simulink model "scheme_w_Adaptive"  (R2025a)
settings: Solver=ode4  StartTime=0.0  StopTime=36  FixedStep=0.001  RelTol=1e-3
values from neighbouring files (symbols this model uses):
  x0 = zeros(14, 1)    [Planning_Sim.m]
undefined symbols (not defined in the file or in its folder): alpha, Am_x, Am_y, Am_z, B_pitch, B_roll, B_spin, beta, Bm_x, Bm_y, Bm_z, Cm_x, Cm_y, Dm_x, Dm_y, gamma, p, Px, Py, Pz
settings Model: Creator=chiar_zjcy1by  LastModifiedBy=chiar_zjcy1by
settings SolverCC: ZeroCrossAlgorithm=Adaptive
settings DebuggingCC: IgnoredZcDiagnostic=none

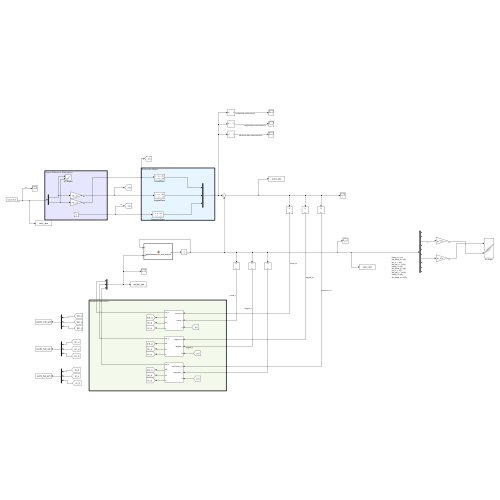
[thumbnail: Simulink's stored preview of the top-level diagram]
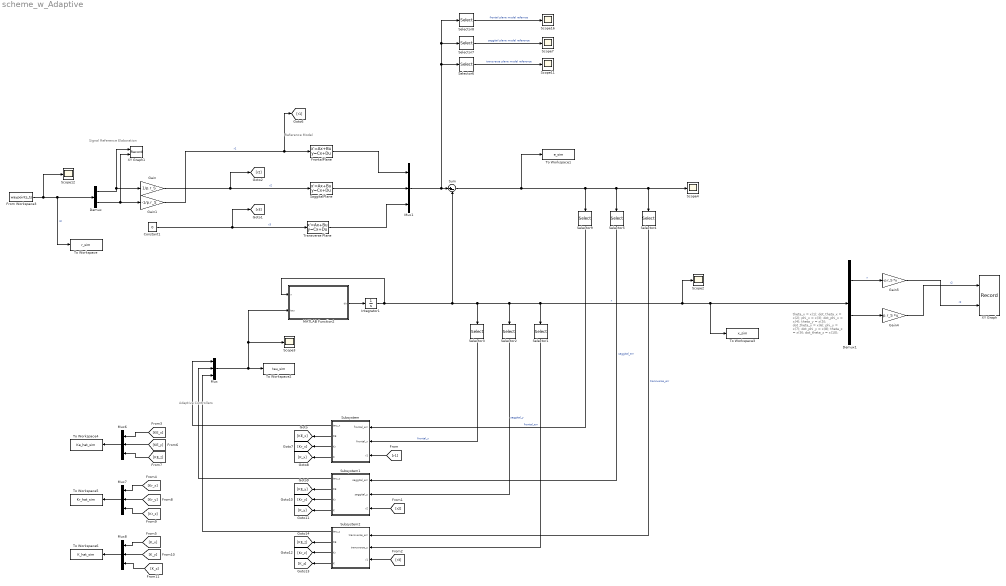
== system scheme_w_Adaptive ==
  note: Signal Reference Elaboration
  note: Reference Model
  note: Adaptive Controllers
  note: theta_x = x(1);
      | dot_theta_x = x(2);
      | phi_x = x(3);
      | dot_phi_x = x(4);
      | theta_y = x(5);
      | dot_theta_y = x(6);
      | phi_y = x(7);
      | dot_phi_y = x(8);
      | theta_z = x(9);
      | dot_theta_z = x(10);
  Constant1 : Constant  Value=0
  Demux : Demux  Outputs=2
  Demux1 : Demux  Outputs=10
  From Workspace3 : FromWorkspace  VariableName=waypoints_ts  SampleTime=0.01  OutputAfterFinalValue=Holding final value
  FrontalPlane : StateSpace  A=Am_x  B=Bm_x  C=Cm_x  D=Dm_x  InitialCondition=x0(1:4)
  Gain : Gain  Gain=1/p.r_S
  Gain1 : Gain  Gain=-1/p.r_S
  Gain4 : Gain  Gain=p.r_S  Multiplication=Matrix(K*u)
  Gain5 : Gain  Gain=-p.r_S  Multiplication=Matrix(K*u)
  Integrator1 : Integrator  InitialCondition=x0
  MATLAB Function2 : MATLAB Function  TreatAsAtomicUnit=on
  Mux{,1,6..8} (5 alike) : Mux  Inputs=3
  SaggitalPlane : StateSpace  A=Am_y  B=Bm_y  C=Cm_y  D=Dm_y  InitialCondition=x0(5:8)
  Scope{2..4,7,11..12,16} (7 alike) : Scope
      Scope11 settings: ActiveDisplayYMinimum=-1  ActiveDisplayYMaximum=1  DataLoggingVariableName=ScopeData19
      Scope12 settings: ActiveDisplayYMinimum=-0.55116650388768529  ActiveDisplayYMaximum=4.9604985349891688  DataLoggingVariableName=ScopeData20  DataLoggingSaveFormat=Array
      Scope16 settings: ActiveDisplayYMinimum=-1.561360729010373  ActiveDisplayYMaximum=5.3735398831765027  DataLoggingVariableName=ScopeData25
      Scope2 settings: ActiveDisplayYMinimum=-2.4855756069167088  ActiveDisplayYMaximum=12.484215788226109
      Scope3 settings: ActiveDisplayYMinimum=-105.04370048469272  ActiveDisplayYMaximum=581.33162472829531  DataLoggingVariableName=ScopeData9
      Scope4 settings: ActiveDisplayYMinimum=-19.49948502397293  ActiveDisplayYMaximum=7.9410058565728949  DataLoggingVariableName=ScopeData2
      Scope7 settings: ActiveDisplayYMinimum=-5.03194060462366  ActiveDisplayYMaximum=39.484259056634677  DataLoggingVariableName=ScopeData13
  Selector1 : Selector  InputPortWidth=10  IndexOptions=Index vector (dialog)  Indices=[9 10]  OutputSizes=1
  Selector2 : Selector  InputPortWidth=10  IndexOptions=Index vector (dialog)  Indices=[5 6 7 8]  OutputSizes=1
  Selector3 : Selector  InputPortWidth=10  IndexOptions=Index vector (dialog)  Indices=[1 2 3 4]  OutputSizes=1
  Selector4 : Selector  InputPortWidth=10  IndexOptions=Index vector (dialog)  Indices=[9 10]  OutputSizes=1
  Selector5 : Selector  InputPortWidth=10  IndexOptions=Index vector (dialog)  Indices=[5 6 7 8]  OutputSizes=1
  Selector6 : Selector  InputPortWidth=10  IndexOptions=Index vector (dialog)  Indices=[9 10]  OutputSizes=1
  Selector7 : Selector  InputPortWidth=10  IndexOptions=Index vector (dialog)  Indices=[5 6 7 8]  OutputSizes=1
  Selector8 : Selector  InputPortWidth=10  IndexOptions=Index vector (dialog)  Indices=[1 2 3 4]  OutputSizes=1
  Selector9 : Selector  InputPortWidth=10  IndexOptions=Index vector (dialog)  Indices=[1 2 3 4]  OutputSizes=1
  Subsystem : Subsystem
  Subsystem1 : Subsystem
  Subsystem2 : Subsystem
  Sum : Sum  Inputs=|+-
  To Workspace : ToWorkspace  VariableName=r_sim  SaveFormat=Structure With Time  SampleTime=-1
  To Workspace1 : ToWorkspace  VariableName=e_sim  SaveFormat=Structure With Time  SampleTime=-1
  To Workspace2 : ToWorkspace  VariableName=tau_sim  SaveFormat=Structure With Time  SampleTime=-1
  To Workspace3 : ToWorkspace  VariableName=x_sim  SaveFormat=Structure With Time  SampleTime=-1
  To Workspace4 : ToWorkspace  VariableName=Ke_hat_sim  SaveFormat=Structure With Time  SampleTime=-1
  To Workspace5 : ToWorkspace  VariableName=Kr_hat_sim  SaveFormat=Structure With Time  SampleTime=-1
  To Workspace6 : ToWorkspace  VariableName=K_hat_sim  SaveFormat=Structure With Time  SampleTime=-1
  Transverse Plane : StateSpace  A=Am_z  B=Bm_z  C=eye(2)  D=zeros(2,1)  InitialCondition=x0(9:end)
  XY Graph : Record  NumPorts=2.0  FileSettingsInternal="{\"entries\":[{\"content\":{\"excelSettings\":{\"content\":{},\"type\":\"Streamout.ExcelSettings\"},\"parquetSettings\":{\"content\":{},\"type\":\"Streamout.ParquetSettings\"}},\"type\":\"Streamout.FileSettingStorage\",\"uuid\":\"\"}],\"packageUris\":[\"http:\\/\\/schema.mathworks.com\\/mf0\\/streamout_blocks\\/R2020a\"],\"version\":\"1.0\"}"  FrameSettings=[0, 0]  Layout=[1 1]  SignalsInternal="{\"entries\":[{\"content\":{\"signals\":[{\"content\":{\"blockPath\":[],\"dimensions\":[1,1],\"domain\":\"\",\"lineColor\":\"#a2142f\",\"plots\":[ 1 ],\"port\":1,\"signalID\":1,\"signalName\":\"r2\"},\"type\":\"RecordBlkView.Signal\",\"uuid\":\"\"},{\"content\":{\"blockPath\":[],\"dimensions\":[1,1],\"domain\":\"\",\"lineColor\":\"#139fff\",\"plots\":[ 1 ],\"port\":2,\"signalID\":2,\"signalName\":\"r2\"},\"type\":\"RecordBlkView.Signal\",\"uuid\":\"\"}]},\"type\":\"RecordBlkView.InputSignals\",\"uuid\":\"\"}],\"packageUris\":[\"http:\\/\\/schema.mathworks.com\\/mf0\\/streamout_blocks\\/R2020a\"],\"version\":\"1.0\"}"  VisualizationBindings="{\"xyplotplugin\":{\"info\":[{\"series\":[{\"bindingParametersList\":[{\"parameter\":\"X-Axis\",\"signalID\":1,\"signalName\":\"r2\"},{\"parameter\":\"Y-Axis\",\"signalID\":2,\"signalName\":\"r2\"}],\"seriesID\":0}],\"subplotID\":1}]}}"  CompatibilityTag=XY
  XY Graph1 : Record  NumPorts=2.0  FileSettingsInternal="{\"entries\":[{\"content\":{\"excelSettings\":{\"content\":{},\"type\":\"Streamout.ExcelSettings\"},\"parquetSettings\":{\"content\":{},\"type\":\"Streamout.ParquetSettings\"}},\"type\":\"Streamout.FileSettingStorage\",\"uuid\":\"\"}],\"packageUris\":[\"http:\\/\\/schema.mathworks.com\\/mf0\\/streamout_blocks\\/R2020a\"],\"version\":\"1.0\"}"  FrameSettings=[0, 0]  Layout=[1 1]  SignalsInternal="{\"entries\":[{\"content\":{\"signals\":[{\"content\":{\"blockPath\":[],\"dimensions\":[1],\"domain\":\"\",\"lineColor\":\"#a2142f\",\"plots\":[ 1 ],\"port\":1,\"signalID\":1,\"signalName\":\"Demux:1\"},\"type\":\"RecordBlkView.Signal\",\"uuid\":\"\"},{\"content\":{\"blockPath\":[],\"dimensions\":[1],\"domain\":\"\",\"lineColor\":\"#139fff\",\"plots\":[ 1 ],\"port\":2,\"signalID\":2,\"signalName\":\"Demux:2\"},\"type\":\"RecordBlkView.Signal\",\"uuid\":\"\"}]},\"type\":\"RecordBlkView.InputSignals\",\"uuid\":\"\"}],\"packageUris\":[\"http:\\/\\/schema.mathworks.com\\/mf0\\/streamout_blocks\\/R2020a\"],\"version\":\"1.0\"}"  VisualizationBindings="{\"xyplotplugin\":{\"info\":[{\"series\":[{\"bindingParametersList\":[{\"parameter\":\"X-Axis\",\"signalID\":1,\"signalName\":\"Demux:1\"},{\"parameter\":\"Y-Axis\",\"signalID\":2,\"signalName\":\"Demux:2\"}],\"seriesID\":0}],\"subplotID\":1}]}}"  CompatibilityTag=XY
  wires:
  MATLAB Function2/1(dx) -> Integrator1/1
  Integrator1/1 -> MATLAB Function2/1(x), Selector3/1, Selector2/1, Selector1/1, To Workspace3/1, Demux1/1, Scope2/1, Sum/2  "x"
  From Workspace3/1 -> Scope12/1, To Workspace/1, Demux/1  "r3"
  Demux/2 -> Gain1/1, XY Graph1/2
  Demux/1 -> XY Graph1/1, Gain/1
  Gain/1 -> SaggitalPlane/1, [r2]  "r2"
  Gain1/1 -> FrontalPlane/1, [r1]  "r1"
  Transverse Plane/1 -> Mux1/3
  Constant1/1 -> [r3], Transverse Plane/1  "r3"
  Selector8/1 -> Scope16/1  "frontal plane model refernce"
  Selector6/1 -> Scope11/1  "transverse plane model reference"
  Selector7/1 -> Scope7/1  "saggital plane model reference"
  Mux1/1 -> Sum/1, Selector6/1, Selector8/1, Selector7/1
  [r3] -> Subsystem2/3(r1)
  [r2] -> Subsystem1/3(r2)
  [r1] -> Subsystem/3(r1)
  Selector4/1 -> Subsystem2/1(transverse_err)  "transverse_err"
  Selector5/1 -> Subsystem1/1(saggital_err)  "saggital_err"
  Selector1/1 -> Subsystem2/2(transverse_y)
  Selector2/1 -> Subsystem1/2(saggital_y)  "saggital_y"
  Subsystem/1(tau_x) -> Mux/1
  Selector9/1 -> Subsystem/1(frontal_err)  "frontal_err"
  Selector3/1 -> Subsystem/2(frontal_x)  "frontal_x"
  Subsystem2/1(tau_z) -> Mux/3
  Subsystem1/1(tau_y) -> Mux/2
  Sum/1 -> To Workspace1/1, Selector9/1, Selector5/1, Selector4/1, Scope4/1
  Mux/1 -> To Workspace2/1, MATLAB Function2/2(tau), Scope3/1
  Gain5/1 -> XY Graph/2  "r2"
  Gain4/1 -> XY Graph/1  "r2"
  Demux1/7 -> Gain4/1
  Demux1/3 -> Gain5/1  "x"
  FrontalPlane/1 -> Mux1/1
  SaggitalPlane/1 -> Mux1/2
  Mux6/1 -> To Workspace4/1
  Mux7/1 -> To Workspace5/1
  Mux8/1 -> To Workspace6/1
  Subsystem/2(KE) -> [KE_x]
  Subsystem/3(Kr) -> [Kr_x]
  Subsystem/4(K) -> [K_x]
  [KE_x] -> Mux6/1
  [Kr_x] -> Mux7/1
  [K_x] -> Mux8/1
  Subsystem1/2(KE) -> [KE_y]
  Subsystem1/3(Kr) -> [Kr_y]
  Subsystem1/4(K) -> [K_y]
  Subsystem2/4(K) -> [K_z]
  Subsystem2/3(Kr) -> [Kr_z]
  Subsystem2/2(KE) -> [KE_z]
  [KE_y] -> Mux6/2
  [KE_z] -> Mux6/3
  [Kr_y] -> Mux7/2
  [Kr_z] -> Mux7/3
  [K_y] -> Mux8/2
  [K_z] -> Mux8/3

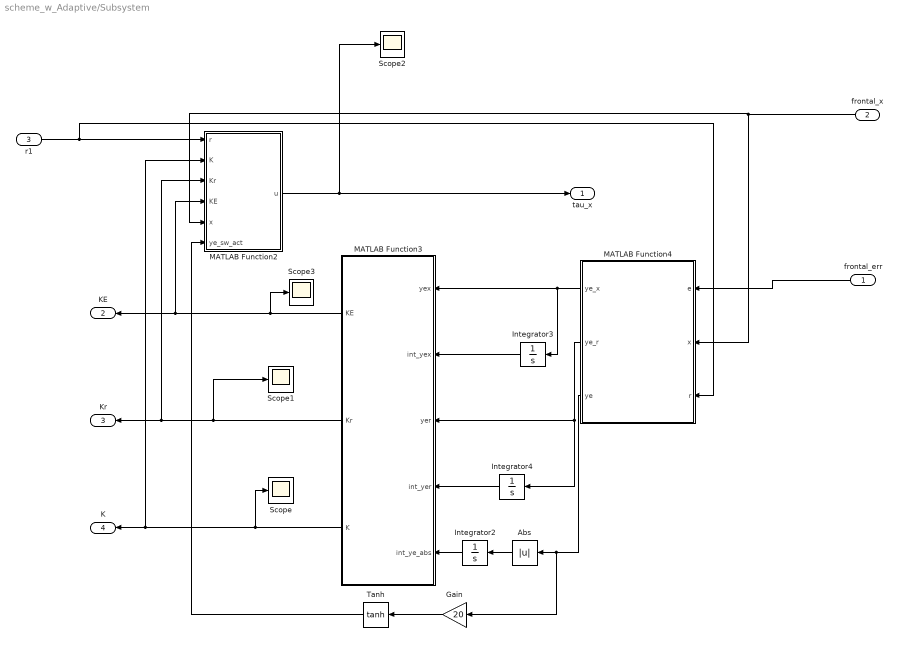
== system scheme_w_Adaptive/Subsystem ==
  frontal_err : Inport
  frontal_x : Inport  Port=2
  r1 : Inport  Port=3
  Abs : Abs  SaturateOnIntegerOverflow=off
  Gain : Gain  Gain=20
  Integrator2 : Integrator
  Integrator3 : Integrator
  Integrator4 : Integrator
  MATLAB Function2 : MATLAB Function  TreatAsAtomicUnit=on
  MATLAB Function3 : MATLAB Function  TreatAsAtomicUnit=on
  MATLAB Function4 : MATLAB Function  TreatAsAtomicUnit=on
  Scope{,1..3} (4 alike) : Scope
      Scope settings: ActiveDisplayYMinimum=-14.804673903534876  ActiveDisplayYMaximum=11.360372956626584  DataLoggingVariableName=ScopeData6
      Scope1 settings: ActiveDisplayYMinimum=-5.521667452338054  ActiveDisplayYMaximum=5.1005284890822695  DataLoggingVariableName=ScopeData7
      Scope2 settings: ActiveDisplayYMinimum=-1  ActiveDisplayYMaximum=1  DataLoggingVariableName=ScopeData8
      Scope3 settings: ActiveDisplayYMinimum=-0.58024840891684848  ActiveDisplayYMaximum=5.2222356802516376  DataLoggingVariableName=ScopeData12
  Tanh : Trigonometry  Operator=tanh
  tau_x : Outport
  KE : Outport  Port=2
  Kr : Outport  Port=3
  K : Outport  Port=4
  wires:
  MATLAB Function2/1(u) -> tau_x/1, Scope2/1
  frontal_err/1 -> MATLAB Function4/1(e)
  Integrator4/1 -> MATLAB Function3/4(int_yer)
  Integrator3/1 -> MATLAB Function3/2(int_yex)
  MATLAB Function3/3(K) -> K/1, MATLAB Function2/2(K), Scope/1
  r1/1 -> MATLAB Function2/1(r), MATLAB Function4/3(r)
  frontal_x/1 -> MATLAB Function4/2(x), MATLAB Function2/5(x)
  Integrator2/1 -> MATLAB Function3/5(int_ye_abs)
  MATLAB Function4/2(ye_r) -> Integrator4/1, MATLAB Function3/3(yer)
  MATLAB Function4/1(ye_x) -> MATLAB Function3/1(yex), Integrator3/1
  MATLAB Function4/3(ye) -> Gain/1, Abs/1
  MATLAB Function3/1(KE) -> KE/1, MATLAB Function2/4(KE), Scope3/1
  MATLAB Function3/2(Kr) -> Kr/1, MATLAB Function2/3(Kr), Scope1/1
  Abs/1 -> Integrator2/1
  Tanh/1 -> MATLAB Function2/6(ye_sw_act)
  Gain/1 -> Tanh/1

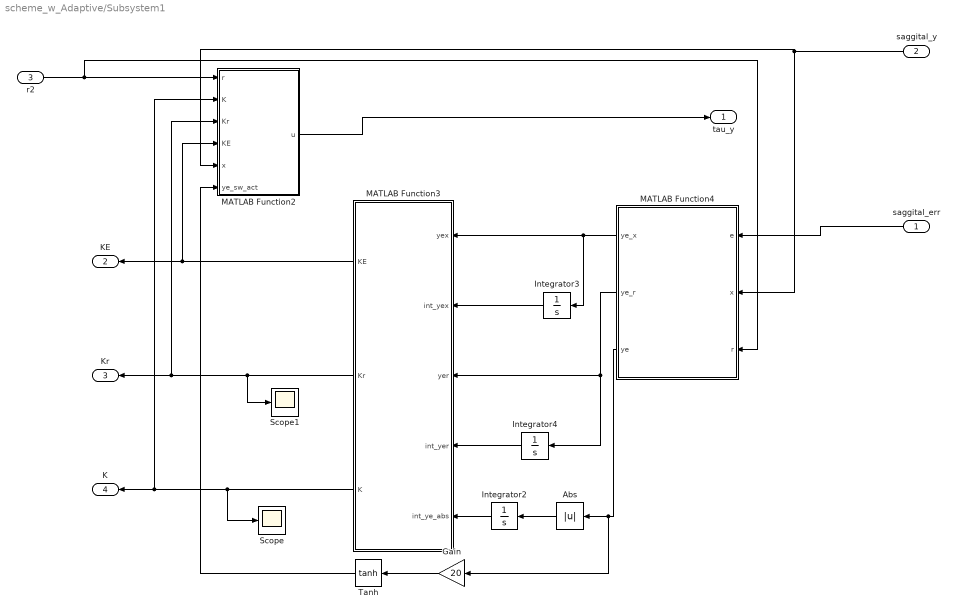
== system scheme_w_Adaptive/Subsystem1 ==
  saggital_err : Inport
  saggital_y : Inport  Port=2
  r2 : Inport  Port=3
  Abs : Abs  SaturateOnIntegerOverflow=off
  Gain : Gain  Gain=20
  Integrator2 : Integrator
  Integrator3 : Integrator
  Integrator4 : Integrator
  MATLAB Function2 : MATLAB Function  TreatAsAtomicUnit=on
  MATLAB Function3 : MATLAB Function  TreatAsAtomicUnit=on
  MATLAB Function4 : MATLAB Function  TreatAsAtomicUnit=on
  Scope : Scope
      settings: ActiveDisplayYMinimum=-11.265590181638307  ActiveDisplayYMaximum=11.140268912066722  DataLoggingVariableName=ScopeData15
  Scope1 : Scope
      settings: ActiveDisplayYMinimum=-1.1237910832802247  ActiveDisplayYMaximum=0.19750652048632228  DataLoggingVariableName=ScopeData16
  Tanh : Trigonometry  Operator=tanh
  tau_y : Outport
  KE : Outport  Port=2
  Kr : Outport  Port=3
  K : Outport  Port=4
  wires:
  MATLAB Function2/1(u) -> tau_y/1
  MATLAB Function3/3(K) -> K/1, MATLAB Function2/2(K), Scope/1
  MATLAB Function3/2(Kr) -> Kr/1, MATLAB Function2/3(Kr), Scope1/1
  MATLAB Function3/1(KE) -> KE/1, MATLAB Function2/4(KE)
  MATLAB Function4/3(ye) -> Gain/1, Abs/1
  MATLAB Function4/1(ye_x) -> Integrator3/1, MATLAB Function3/1(yex)
  MATLAB Function4/2(ye_r) -> MATLAB Function3/3(yer), Integrator4/1
  Integrator2/1 -> MATLAB Function3/5(int_ye_abs)
  saggital_y/1 -> MATLAB Function2/5(x), MATLAB Function4/2(x)
  r2/1 -> MATLAB Function4/3(r), MATLAB Function2/1(r)
  Integrator3/1 -> MATLAB Function3/2(int_yex)
  Integrator4/1 -> MATLAB Function3/4(int_yer)
  saggital_err/1 -> MATLAB Function4/1(e)
  Abs/1 -> Integrator2/1
  Tanh/1 -> MATLAB Function2/6(ye_sw_act)
  Gain/1 -> Tanh/1

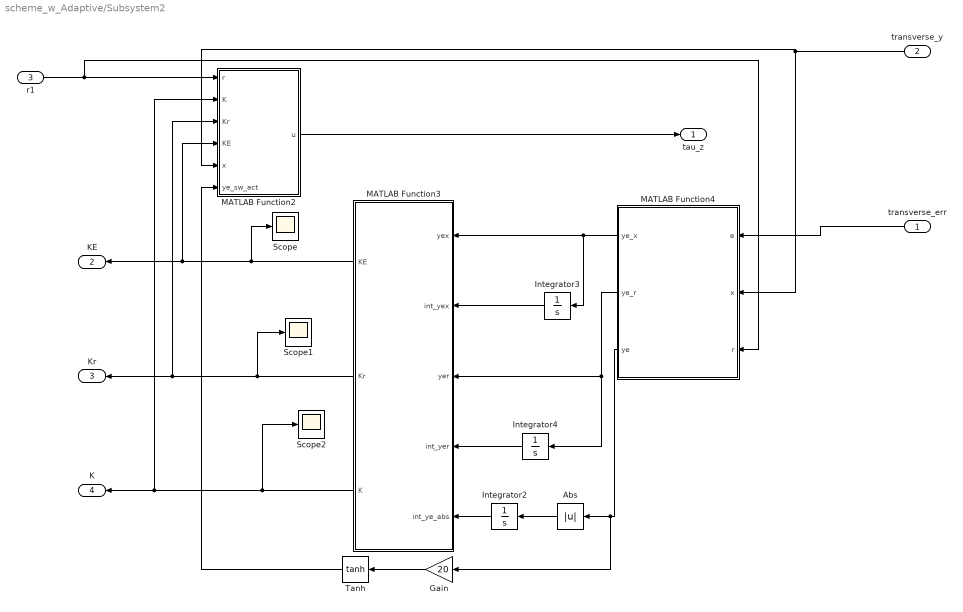
== system scheme_w_Adaptive/Subsystem2 ==
  transverse_err : Inport
  transverse_y : Inport  Port=2
  r1 : Inport  Port=3
  Abs : Abs  SaturateOnIntegerOverflow=off
  Gain : Gain  Gain=20
  Integrator2 : Integrator
  Integrator3 : Integrator
  Integrator4 : Integrator
  MATLAB Function2 : MATLAB Function  TreatAsAtomicUnit=on
  MATLAB Function3 : MATLAB Function  TreatAsAtomicUnit=on
  MATLAB Function4 : MATLAB Function  TreatAsAtomicUnit=on
  Scope : Scope
      settings: ActiveDisplayYMinimum=-1  ActiveDisplayYMaximum=1
  Scope1 : Scope
      settings: ActiveDisplayYMinimum=-1  ActiveDisplayYMaximum=1  DataLoggingVariableName=ScopeData2
  Scope2 : Scope
      settings: ActiveDisplayYMinimum=-1  ActiveDisplayYMaximum=1  DataLoggingVariableName=ScopeData3
  Tanh : Trigonometry  Operator=tanh
  tau_z : Outport
  KE : Outport  Port=2
  Kr : Outport  Port=3
  K : Outport  Port=4
  wires:
  MATLAB Function2/1(u) -> tau_z/1
  transverse_err/1 -> MATLAB Function4/1(e)
  Integrator4/1 -> MATLAB Function3/4(int_yer)
  Integrator3/1 -> MATLAB Function3/2(int_yex)
  MATLAB Function3/3(K) -> K/1, MATLAB Function2/2(K), Scope2/1
  r1/1 -> MATLAB Function2/1(r), MATLAB Function4/3(r)
  transverse_y/1 -> MATLAB Function4/2(x), MATLAB Function2/5(x)
  Integrator2/1 -> MATLAB Function3/5(int_ye_abs)
  MATLAB Function4/2(ye_r) -> Integrator4/1, MATLAB Function3/3(yer)
  MATLAB Function4/1(ye_x) -> MATLAB Function3/1(yex), Integrator3/1
  MATLAB Function3/1(KE) -> KE/1, MATLAB Function2/4(KE), Scope/1
  MATLAB Function3/2(Kr) -> Kr/1, MATLAB Function2/3(Kr), Scope1/1
  Abs/1 -> Integrator2/1
  MATLAB Function4/3(ye) -> Gain/1, Abs/1
  Tanh/1 -> MATLAB Function2/6(ye_sw_act)
  Gain/1 -> Tanh/1

== matlab function scheme_w_Adaptive/Subsystem2/MATLAB Function2 ==
  data: r input; K input; Kr input; KE input; u output; x input; ye_sw_act input
function u = controller(r, K,Kr,KE,x,ye_sw_act)
u = K*x+Kr*r+KE*ye_sw_act;

== matlab function scheme_w_Adaptive/Subsystem2/MATLAB Function3 ==
  data: KE output; Kr output; yex input; K output; int_yex input; yer input; int_yer input; int_ye_abs input; alpha parameter; beta parameter; gamma parameter
function [KE, Kr, K] = adapt_law(yex, int_yex, yer, int_yer, int_ye_abs, alpha, beta, gamma)

    K= alpha* int_yex + beta*yex;
    Kr= alpha * int_yer + beta*yer;
    KE = gamma * int_ye_abs;

end

== matlab function scheme_w_Adaptive/Subsystem2/MATLAB Function4 ==
  data: ye_x output; ye_r output; e input; ye output; x input; r input; B_spin parameter; Pz parameter
function [ye_x, ye_r,ye] = y_e_computation(e, x, r, B_spin, Pz)
ye = B_spin'*Pz*e;
ye_x = ye*x';
ye_r = ye*r';

== matlab function scheme_w_Adaptive/MATLAB Function2 ==
  data: x input; p parameter; tau input; dx output
function dx = stateDerivative3D_with_exforce(x, p, tau)
    % MODIFICATION 1: The function now accepts a 4th argument, 'wrench_ext',
    % which is a vector containing the external forces and torques from Simulink.


    % Unpack state vector (10 elements)
    theta_x = x(1); 
    dot_theta_x = x(2);
    % phi_x = x(3); % Not needed for dynamicsù
    dot_phi_x   = x(4);

    theta_y = x(5); 
    dot_theta_y = x(6);
    % phi_y   = x(7); % Not needed for dynamics
    dot_phi_y   = x(8);

    theta_z = x(9); 
    dot_theta_z = x(10);

    % Unpack input torques
    tau_x = tau(1);
    tau_y = tau(2);
    tau_z = tau(3);

    %  % Unpack the external wrench vector from the new input ---
    % % Expected order: [F_px, F_py, F_pz, tau_px, tau_py]
    % F_px   = wrench_ext(1);
    % F_py   = wrench_ext(2);
    % F_pz   = wrench_ext(3);
    % tau_px = wrench_ext(4);
    % tau_py = wrench_ext(5);
    % tau_pz = wrench_ext(6);

    % --- Prepare arguments for auto-generated functions ---
    % Create separate parameter vectors for each plane, now including h_app
    % Note: I_Ux is for roll, I_Uy is for pitch.
    params_arg_roll = [p.m_U, p.I_Uy, p.I_Ux, p.l_U, p.m_S, p.I_S, p.r_S, p.g, p.b_theta, p.b_phi, p.h_app];
    params_arg_pitch = [p.m_U,p.I_Uy, p.I_Ux, p.l_U, p.m_S, p.I_S, p.r_S, p.g, p.b_theta, p.b_phi, p.h_app];

    % external_vars_x = [F_py, F_pz, tau_px]; % For Roll dynamics
    % external_vars_y = [F_px, F_pz, tau_py]; % For Pitch dynamics

    % --- X-Z Plane (Roll) Dynamics ---
    states_arg_x = [theta_x, dot_theta_x, dot_phi_x];
    inputs_arg_x = [tau_x];
    ddot_theta_x = autogen_ddot_theta_x(states_arg_x, inputs_arg_x, params_arg_roll);
    ddot_phi_x   = autogen_ddot_phi_x(states_arg_x, inputs_arg_x, params_arg_roll);


    % --- Y-Z Plane (Pitch) Dynamics ---
    states_arg_y = [theta_y, dot_theta_y, dot_phi_y];
    inputs_arg_y = [tau_y];
    ddot_theta_y = autogen_ddot_theta_y(states_arg_y, inputs_arg_y, params_arg_pitch);
    ddot_phi_y   = autogen_ddot_phi_y(states_arg_y, inputs_arg_y, params_arg_pitch);

    % --- Transversal Plane Dynamics (Yaw) ---
    % external forces at the center of the top surface are assumed not to produce yaw torque.
    ddot_theta_z = (tau_z - p.fz * dot_theta_z) / p.Iz;

    % --- Assemble the state derivative vector dx ---
    dx = [
        dot_theta_x;    % dx(1) = d(theta_x)/dt
        ddot_theta_x;   % dx(2) = d(dot_theta_x)/dt
        dot_phi_x;      % dx(3) = d(phi_x)/dt
        ddot_phi_x;     % dx(4) = d(dot_phi_x)/dt

        dot_theta_y;    % dx(5) = d(theta_y)/dt 
        ddot_theta_y;   % dx(6) = d(dot_theta_y)/dt
        dot_phi_y;      % dx(7) = d(phi_y)/dt
        ddot_phi_y;     % dx(8)= d(dot_phi_y)/dt

        dot_theta_z;    % dx(9) = d(theta_z)/dt
        ddot_theta_z;   % dx(10) = d(dot_theta_z)/dt
    ];
end

% function dx = stateDerivative3D_generated(x, tau, p)
%     % SW was assumed to not spin relative to the ground
% 
%     % Unpack state vector (10 elements)
%     theta_x = x(1); 
%     dot_theta_x = x(2);
%     % phi_x = x(3); % Not needed for dynamicsù
%     dot_phi_x   = x(4);
% 
%     theta_y = x(5); 
%     dot_theta_y = x(6);
%     % phi_y   = x(7); % Not needed for dynamics
%     dot_phi_y   = x(8);
% 
%     theta_z = x(9); 
%     dot_theta_z = x(10);
% 
%     % Unpack input torques
%     tau_x = tau(1);
%     tau_y = tau(2);
%     tau_z = tau(3);
% 
%     % --- Prepare arguments for auto-generated functions ---
%     % Argument list for parameters (order MUST match the generator script)
%     params_arg = [p.m_U, p.I_Uy, p.I_Ux, p.l_U, p.m_S, p.I_S, p.r_S, p.g, p.b_theta, p.b_phi];
% 
%     % --- X-Z Plane (Roll) Dynamics ---
%     states_arg_x = [theta_x, dot_theta_x, dot_phi_x];
%     inputs_arg_x = [tau_x];
%     ddot_theta_x = autogen_ddot_theta_x(states_arg_x, inputs_arg_x, params_arg);
%     ddot_phi_x   = autogen_ddot_phi_x(states_arg_x, inputs_arg_x, params_arg);
% 
%     % --- Y-Z Plane (Pitch) Dynamics ---
%     states_arg_y = [theta_y, dot_theta_y, dot_phi_y];
%     inputs_arg_y = [tau_y];
%     ddot_theta_y = autogen_ddot_theta_y(states_arg_y, inputs_arg_y, params_arg);
%     ddot_phi_y   = autogen_ddot_phi_y(states_arg_y, inputs_arg_y, params_arg);
% 
%     % --- Transversal Plane Dynamics (Yaw) ---
%     % Using the simple decoupled model from your original script
%     ddot_theta_z = (tau_z - p.fz * dot_theta_z) / p.Iz;
% 
%     % --- Assemble the state derivative vector dx ---
%     dx = [
%         dot_theta_x;    % dx(1) = d(theta_x)/dt
%         ddot_theta_x;   % dx(2) = d(dot_theta_x)/dt
%         dot_phi_x;      % dx(3) = d(phi_x)/dt
%         ddot_phi_x;     % dx(4) = d(dot_phi_x)/dt
% 
%         dot_theta_y;    % dx(5) = d(theta_y)/dt 
%         ddot_theta_y;   % dx(6) = d(dot_theta_y)/dt
%         dot_phi_y;      % dx(7) = d(phi_y)/dt
%         ddot_phi_y;     % dx(8)= d(dot_phi_y)/dt
% 
%         dot_theta_z;    % dx(9) = d(theta_z)/dt
%         ddot_theta_z;   % dx(10) = d(dot_theta_z)/dt
%     ];
% end

== matlab function scheme_w_Adaptive/Subsystem/MATLAB Function4 ==
  data: ye_x output; ye_r output; e input; ye output; x input; r input; B_roll parameter; Px parameter
function [ye_x, ye_r,ye] = y_e_computation(e, x, r, B_roll, Px)
ye = B_roll'*Px*e;
ye_x = ye*x';
ye_r = ye*r';

== matlab function scheme_w_Adaptive/Subsystem/MATLAB Function2 ==
  data: r input; K input; Kr input; KE input; u output; x input; ye_sw_act input
function u = controller(r, K,Kr,KE,x,ye_sw_act)
u = K*x+Kr*r+KE*ye_sw_act;

== matlab function scheme_w_Adaptive/Subsystem/MATLAB Function3 ==
  data: KE output; Kr output; yex input; K output; int_yex input; yer input; int_yer input; int_ye_abs input; alpha parameter; beta parameter; gamma parameter
function [KE, Kr, K] = adapt_law(yex, int_yex, yer, int_yer, int_ye_abs, alpha, beta, gamma)
     
    K= alpha* int_yex + beta*yex;
    Kr= alpha * int_yer + beta*yer;
    KE = gamma * int_ye_abs;

end

== matlab function scheme_w_Adaptive/Subsystem1/MATLAB Function2 ==
  data: r input; K input; Kr input; KE input; u output; x input; ye_sw_act input
function u = controller(r, K,Kr,KE,x,ye_sw_act)
u = K*x+Kr*r+KE*ye_sw_act;

== matlab function scheme_w_Adaptive/Subsystem1/MATLAB Function3 ==
  data: KE output; Kr output; yex input; K output; int_yex input; yer input; int_yer input; int_ye_abs input; alpha parameter; beta parameter; gamma parameter
function [KE, Kr, K] = adapt_law(yex, int_yex, yer, int_yer, int_ye_abs, alpha, beta, gamma)
    
    K= alpha* int_yex + beta*yex;
    Kr= alpha * int_yer + beta*yer;
    KE = gamma * int_ye_abs;
    

end

== matlab function scheme_w_Adaptive/Subsystem1/MATLAB Function4 ==
  data: ye_x output; ye_r output; e input; ye output; x input; r input; B_pitch parameter; Py parameter
function [ye_x, ye_r,ye] = y_e_computation(e, x, r, B_pitch, Py)
ye = B_pitch'*Py*e;
ye_x = ye*x';
ye_r = ye*r';
